simulink model "modelo"  (R2020b)
settings: Solver=VariableStepAuto  StartTime=0.0  StopTime=205.1*6  FixedStep=1e-9  RelTol=1e-3
values from neighbouring files (symbols this model uses):
  Pd = 40    [simulacion_qam.m]    (also in simulacioon.m)
libraries: dsparch4 x1
settings Model: Creator=Mateo  LastModifiedBy=Mateo
settings DataIOCC: ReturnWorkspaceOutputs=off

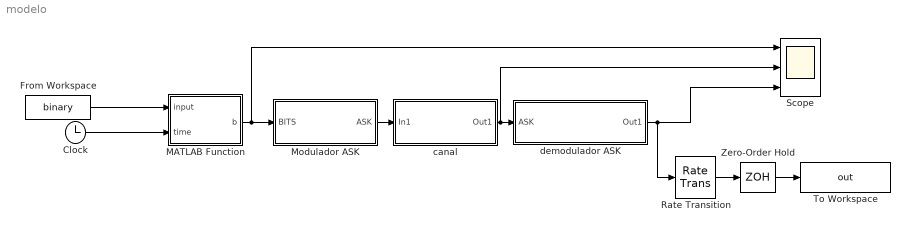
== system modelo ==
  Clock : Clock
  From Workspace : FromWorkspace  VariableName=binary
  MATLAB Function : MATLAB Function  TreatAsAtomicUnit=on
  Modulador ASK : Subsystem
  Rate Transition : RateTransition
  Scope : Scope  NumInputPorts=3
  To Workspace : ToWorkspace  VariableName=out  SaveFormat=Timeseries  SampleTime=-1
  Zero-Order Hold : ZeroOrderHold  SampleTime=6
  canal : Subsystem
  demodulador ASK : Subsystem
  wires:
  From Workspace/1 -> MATLAB Function/1(input)
  Clock/1 -> MATLAB Function/2(time)
  MATLAB Function/1(b) -> Modulador ASK/1(BITS), Scope/1
  demodulador ASK/1(Out1) -> Rate Transition/1, Scope/3
  Rate Transition/1 -> Zero-Order Hold/1
  Zero-Order Hold/1 -> To Workspace/1
  Modulador ASK/1(ASK) -> canal/1(In1)
  canal/1(Out1) -> Scope/2, demodulador ASK/1(ASK)

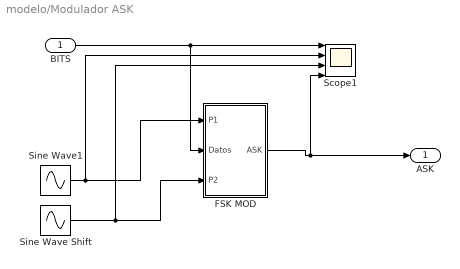
== system modelo/Modulador ASK ==
  BITS : Inport
  FSK MOD : Subsystem
  Scope1 : Scope  NumInputPorts=4
  Sine Wave Shift : Sin  SineType=Sample based  Amplitude=0.5  Frequency=2*10*pi  Phase=-pi  Samples=50  SampleTime=1/20
  Sine Wave1 : Sin  SineType=Sample based  Amplitude=2  Frequency=2*10*pi  Samples=50  SampleTime=1/20
  ASK : Outport
  wires:
  BITS/1 -> Scope1/1, FSK MOD/2(Datos)
  Sine Wave1/1 -> Scope1/2, FSK MOD/1(P1)
  Sine Wave Shift/1 -> Scope1/3, FSK MOD/3(P2)
  FSK MOD/1(ASK) -> Scope1/4, ASK/1

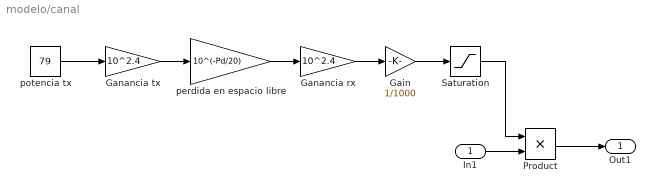
== system modelo/canal ==
  In1 : Inport
  Gain : Gain  Gain=1/1000
  Ganancia rx : Gain  Gain=10^2.4
  Ganancia tx : Gain  Gain=10^2.4
  Product : Product
  Saturation : Saturate  UpperLimit=1  LowerLimit=0
  perdida en espacio libre : Gain  Gain=10^(-Pd/20)
  potencia tx : Constant  Value=79
  Out1 : Outport
  wires:
  potencia tx/1 -> Ganancia tx/1
  Ganancia tx/1 -> perdida en espacio libre/1
  perdida en espacio libre/1 -> Ganancia rx/1
  Product/1 -> Out1/1
  Saturation/1 -> Product/1
  In1/1 -> Product/2
  Ganancia rx/1 -> Gain/1
  Gain/1 -> Saturation/1

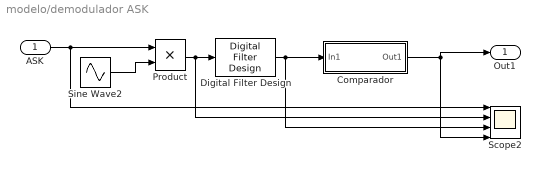
== system modelo/demodulador ASK ==
  ASK : Inport
  Comparador : Subsystem
  Digital Filter Design : dsparch4/Digital Filter Design  mwdsp_browser_bugfix_var=off
  Product : Product  RndMeth=Zero
  Scope2 : Scope  NumInputPorts=4
  Sine Wave2 : Sin  SineType=Sample based  Frequency=2*10*pi  Samples=50  SampleTime=1/20
  Out1 : Outport
  wires:
  ASK/1 -> Scope2/1, Product/1
  Sine Wave2/1 -> Product/2
  Product/1 -> Digital Filter Design/1, Scope2/2
  Digital Filter Design/1 -> Scope2/3, Comparador/1(In1)
  Comparador/1(Out1) -> Scope2/4, Out1/1

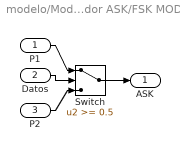
== system modelo/Modulador ASK/FSK MOD ==
  P1 : Inport
  Datos : Inport  Port=2
  P2 : Inport  Port=3
  Switch : Switch  Threshold=0.5
  ASK : Outport
  wires:
  P1/1 -> Switch/1
  Datos/1 -> Switch/2
  Switch/1 -> ASK/1
  P2/1 -> Switch/3

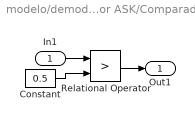
== system modelo/demodulador ASK/Comparador ==
  In1 : Inport
  Constant : Constant  Value=0.5
  Relational Operator : RelationalOperator  Operator=>  OutDataTypeStr=boolean  RndMeth=Nearest
  Out1 : Outport
  wires:
  Constant/1 -> Relational Operator/2
  In1/1 -> Relational Operator/1
  Relational Operator/1 -> Out1/1

== matlab function modelo/MATLAB Function ==
  data: input input; b output; time input
function b = fcn(input,time)
    b=input(floor(time/6)+1);
end
